simulink model "pid_model_disc"  (Simulink 8.1)
settings: Solver=ode4  StartTime=0.0  StopTime=5000.0  FixedStep=1  RelTol=1e-3
libraries: simulink x1
settings Model: Creator=Avega  LastModifiedBy=Avega
settings DataIOCC: SignalLoggingSaveFormat=Dataset
settings OptimizationCC: ExpressionDepthLimit=128
settings DebuggingCC: FcnCallInpInsideContextMsg=EnableAllAsError
settings GRTTargetCC: CombineOutputUpdateFcns=on  GRTInterface=off

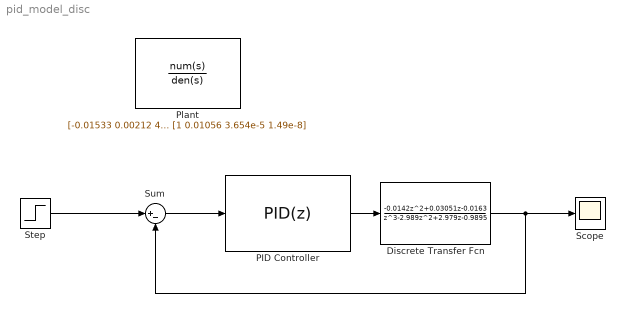
== system pid_model_disc ==
  Discrete Transfer Fcn : DiscreteTransferFcn  Numerator=[-0.0142 0.03051 -0.0163]  Denominator=[1 -2.989 2.979 -0.9895]
  PID Controller : simulink/Continuous/PID Controller  Controller=PID  TimeDomain=Discrete-time  SampleTime=1  IntegratorMethod=Forward Euler  FilterMethod=Forward Euler  Form=Parallel  P=0.185969402279145  I=9.43792899681384e-05  D=26.5437321466882  N=0.293126936672462  InitialConditionSource=internal  InitialConditionForIntegrator=0  InitialConditionForFilter=0  ExternalReset=none  ZeroCross=off  LimitOutput=on  UpperSaturationLimit=1  LowerSaturationLimit=0  LinearizeAsGain=off  AntiWindupMode=clamping  Kb=1  TrackingMode=off  Kt=1  PParamMin=[]  PParamMax=[]  IParamMin=[]  IParamMax=[]  DParamMin=[]  DParamMax=[]  NParamMin=[]  NParamMax=[]  KbParamMin=[]  KbParamMax=[]  KtParamMin=[]  KtParamMax=[]  POutMin=[]  POutMax=[]  IOutMin=[]  IOutMax=[]  DOutMin=[]  DOutMax=[]  NOutMin=[]  NOutMax=[]  KbOutMin=[]  KbOutMax=[]  KtOutMin=[]  KtOutMax=[]  IntegratorOutMin=[]  IntegratorOutMax=[]  FilterOutMin=[]  FilterOutMax=[]  SumOutMin=[]  SumOutMax=[]  SumI1OutMin=[]  SumI1OutMax=[]  SumI2OutMin=[]  SumI2OutMax=[]  SumI3OutMin=[]  SumI3OutMax=[]  SumDOutMin=[]  SumDOutMax=[]  SaturationOutMin=[]  SaturationOutMax=[]  IntegratorContinuousStateAttributes=''  IntegratorStateMustResolveToSignalObject=off  IntegratorRTWStateStorageClass=Auto  FilterContinuousStateAttributes=''  FilterStateMustResolveToSignalObject=off  FilterRTWStateStorageClass=Auto
  Plant : TransferFcn  Numerator=[-0.01533 0.00212 4.827e-6]  Denominator=[1 0.01056 3.654e-5 1.49e-8]
  Scope : Scope
      settings: TimeRange=3000  YMin=-20  YMax=180
  Step : Step  Time=2500  Before=150  After=100  SampleTime=1
  Sum : Sum  Inputs=|+-
  wires:
  Sum/1 -> PID Controller/1
  Step/1 -> Sum/1
  Discrete Transfer Fcn/1 -> Sum/2, Scope/1
  PID Controller/1 -> Discrete Transfer Fcn/1
